simulink model "DaVinci_SimulJ"  (R2023a)
settings: Solver=VariableStepAuto  StartTime=0.0  StopTime=10.0  RelTol=1e-3
libraries: vrlib x7, DaVinci_LibJ x1
settings Model: Creator=ASUS  LastModifiedBy=ASUS

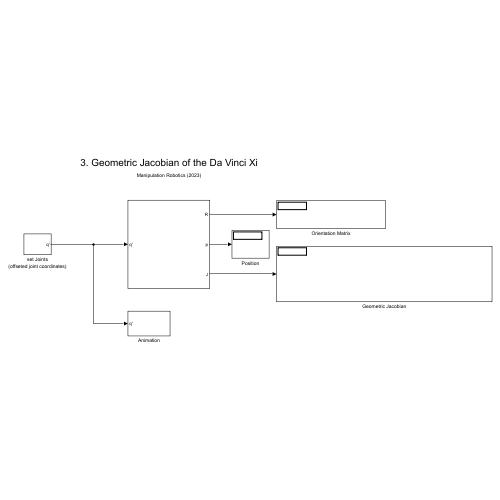
[thumbnail: Simulink's stored preview of the top-level diagram]
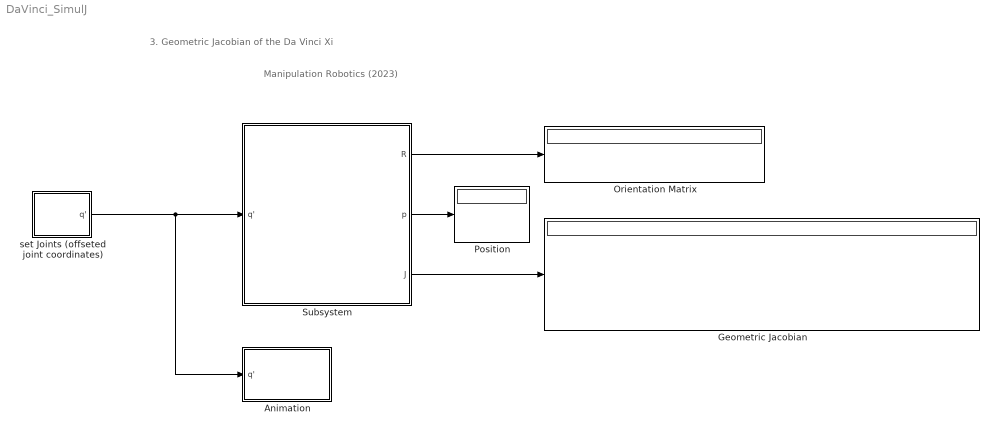
== system DaVinci_SimulJ ==
  note: 3. Geometric Jacobian of the Da Vinci Xi
  note: Manipulation Robotics (2023)
  Animation : Subsystem
  Geometric Jacobian : Display
  Orientation Matrix : Display
  Position : Display
  Subsystem : Subsystem
  set Joints (offseted joint coordinates) : Subsystem  mask{q1=136.800, q2=-68.400, q3=0.660, q4=-50.400, q5=0, q6=0.0}
  wires:
  Subsystem/3(J) -> Geometric Jacobian/1
  Subsystem/2(p) -> Position/1
  Subsystem/1(R) -> Orientation Matrix/1
  set Joints (offseted joint coordinates)/1(q') -> Animation/1(q'), Subsystem/1(q')

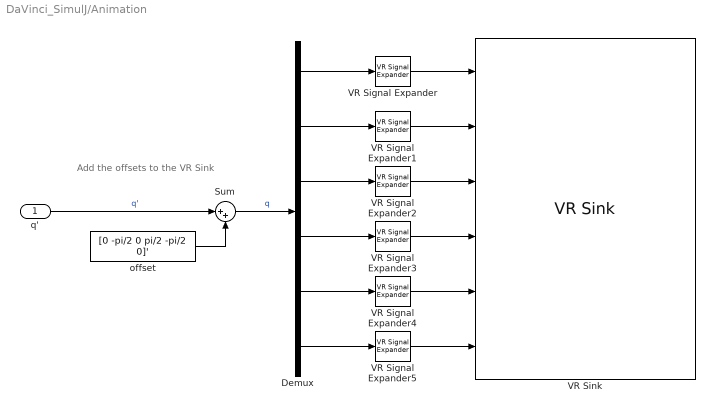
== system DaVinci_SimulJ/Animation ==
  note: Add the offsets to the VR Sink
  q' : Inport
  Demux : Demux  Outputs=6
  Sum : Sum  Inputs=|++
  VR Signal Expander{,1,3..5} (5 alike) : vrlib/VR Signal Expander  outwidth=4  outidx=[4]
  VR Signal Expander2 : vrlib/VR Signal Expander  outwidth=3  outidx=[3]
  VR Sink : vrlib/VR Sink  InstantiateOnLoad=on  SampleTime=-1  ViewEnable=on  RemoteChange=off  RemoteView=off  FieldsWritten=Jt1_DH_dv.rotation.4.1.1.double#Jt2_DH_dv.rotation.4.1.1.double#Jt3_DH_dv.translation.3.1.1.double#Jt4_DH_dv.rotation.4.1.1.double#Jt5_DH_dv.rotation.4.1.1.double#Jt6_DH_dv.rotation.4.1.1.double  WorldFileName=DaVinciFrames.wrl  WorldDescription=Da Vinci Frames  AutoView=on  VideoDimensions=[]  AllowVariableSize=off  FigureProperties="{'Position', 'Name', 'Viewpoint', 'CameraBound', 'CameraDirection', 'CameraPosition', 'CameraUpVector', 'ZoomFactor', 'Antialiasing', 'Headlight', 'Lighting', 'NavPanel', 'Sound', 'StatusBar', 'Stereo3D', 'Stereo3DCameraOffset', 'Stereo3DHIT', 'ToolBar', 'Textures', 'Transparency', 'Triad', 'Wireframe', 'NavZones', 'NavMode', 'NavSpeed', 'CaptureFileFormat', 'CaptureFileName', 'Record2DCompressMethod', 'Record2DCompressQuality', 'Record2D', 'Record2DFileName', 'Record2DFPS'; [7.2033333333333326e+02   9.8666666666666742e+01   5.2500000000000000e+02   4.7833333333333326e+02], 'Da Vinci Frames', 'View 1', 'on', [-2.7798948897595188e-01  -6.1604665392529390e-01   7.3702670521919800e-01], [5.0034199296306081e-01   2.7548856094083285e-01  -4.6461728950164174e+00], [9.6057957170855224e-01  -1.7592067904036524e-01   2.1526449103866996e-01], [1.0000000000000000e+00], 'on', 'on', 'on', 'halfbar', 'on', 'on', 'off', [1.0000000149011612e-01], [0.0000000000000000e+00], 'on', 'on', 'on', 'none', 'off', 'off', 'examine', 'normal', 'tif', '%f_anim_%n.tif', 'auto', [7.5000000000000000e+01], 'off', '%f_anim_%n.avi', 'auto'}"
  offset : Constant  Value=[0 -pi/2 0 pi/2 -pi/2 0]'  VectorParams1D=off
  wires:
  VR Signal Expander2/1 -> VR Sink/3
  offset/1 -> Sum/2
  VR Signal Expander1/1 -> VR Sink/2
  q'/1 -> Sum/1  "q'"
  Sum/1 -> Demux/1  "q"
  Demux/3 -> VR Signal Expander2/1
  Demux/6 -> VR Signal Expander5/1
  VR Signal Expander3/1 -> VR Sink/4
  Demux/1 -> VR Signal Expander/1
  Demux/2 -> VR Signal Expander1/1
  VR Signal Expander4/1 -> VR Sink/5
  Demux/4 -> VR Signal Expander3/1
  Demux/5 -> VR Signal Expander4/1
  VR Signal Expander5/1 -> VR Sink/6
  VR Signal Expander/1 -> VR Sink/1

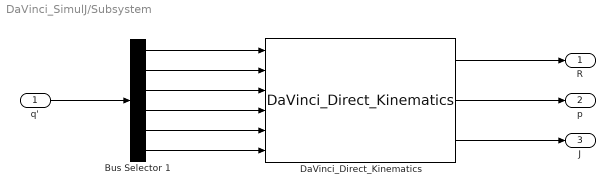
== system DaVinci_SimulJ/Subsystem ==
  q' : Inport
  Bus Selector 1 : Demux  Outputs=6
  DaVinci_Direct_Kinematics : DaVinci_LibJ/DaVinci_Direct_Kinematics  SystemSampleTime=-1  VariantActivationTime=update diagram  Latency=0  AutoFrameSizeCalculation=off
      settings: LibrarySourceBlock=|
      | simulink/User-Defined
      | Functions/MATLAB Function
  R : Outport
  p : Outport  Port=2
  J : Outport  Port=3
  wires:
  Bus Selector 1/2 -> DaVinci_Direct_Kinematics/2
  Bus Selector 1/6 -> DaVinci_Direct_Kinematics/6
  Bus Selector 1/3 -> DaVinci_Direct_Kinematics/3
  Bus Selector 1/1 -> DaVinci_Direct_Kinematics/1
  Bus Selector 1/5 -> DaVinci_Direct_Kinematics/5
  Bus Selector 1/4 -> DaVinci_Direct_Kinematics/4
  DaVinci_Direct_Kinematics/1 -> R/1
  q'/1 -> Bus Selector 1/1
  DaVinci_Direct_Kinematics/2 -> p/1
  DaVinci_Direct_Kinematics/3 -> J/1

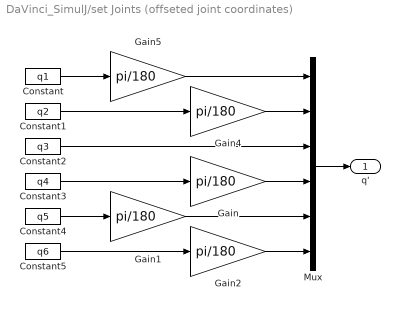
== system DaVinci_SimulJ/set Joints (offseted joint coordinates) ==
  Constant : Constant  Value=q1
  Constant1 : Constant  Value=q2
  Constant2 : Constant  Value=q3
  Constant3 : Constant  Value=q4
  Constant4 : Constant  Value=q5
  Constant5 : Constant  Value=q6
  Gain{,1..2,4..5} (5 alike) : Gain  Gain=pi/180
  Mux : Mux  Inputs=6
  q' : Outport
  wires:
  Gain2/1 -> Mux/6
  Constant1/1 -> Gain4/1
  Constant3/1 -> Gain/1
  Constant5/1 -> Gain2/1
  Mux/1 -> q'/1
  Gain5/1 -> Mux/1
  Gain/1 -> Mux/4
  Gain1/1 -> Mux/5
  Gain4/1 -> Mux/2
  Constant/1 -> Gain5/1
  Constant2/1 -> Mux/3
  Constant4/1 -> Gain1/1
